simulink model "psd_project"  (R2015a)
settings: Solver=ode45  StartTime=0.0  StopTime=10  RelTol=1e-3
libraries: dsparch4 x19, dspvision x13, commchan3 x1
settings Model: Creator=aluno  LastModifiedBy=aluno

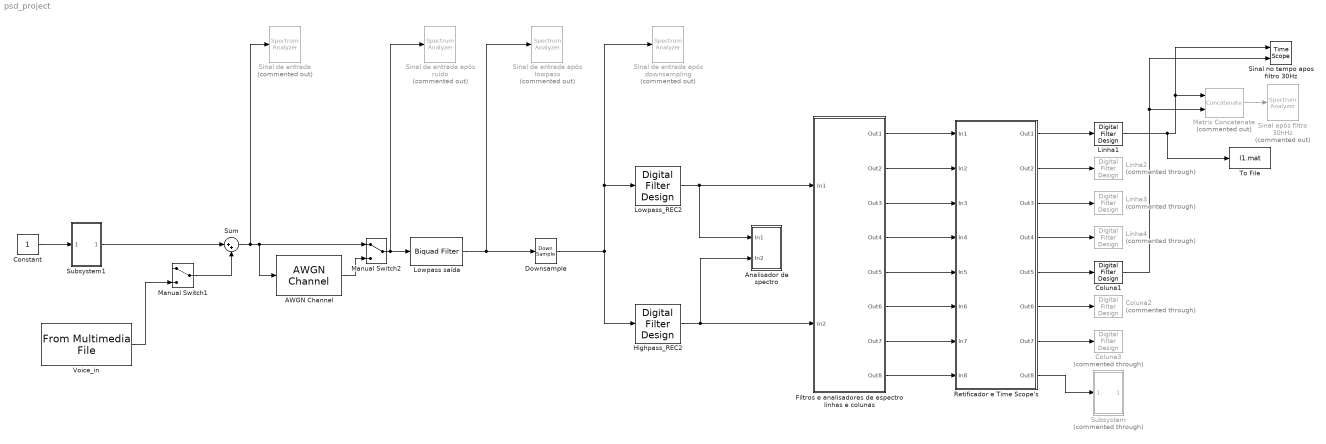
== system psd_project ==
  AWGN Channel : commchan3/AWGN Channel  InputProcessing=Columns as channels (frame based)  seed=67  noiseMode="Signal to noise ratio  (SNR)"  EbNodB=30  EsNodB=10  SNRdB=5  bitsPerSym=1  Ps=1  Tsym=1  variance=1
  Analisador de spectro : Subsystem
  Coluna1 : dsparch4/Digital Filter Design  mwdsp_browser_bugfix_var=off
  Coluna2 : dsparch4/Digital Filter Design  Commented=through  mwdsp_browser_bugfix_var=off
  Coluna3 : dsparch4/Digital Filter Design  Commented=through  mwdsp_browser_bugfix_var=off
  Constant : Constant
  Downsample : DownSample  N=11  RateOptions=Allow multirate processing
  Filtros e analisadores de espectro linhas e colunas : Subsystem
  "Highpass_REC2 " : dsparch4/Digital Filter Design  mwdsp_browser_bugfix_var=off
  Linha1 : dsparch4/Digital Filter Design  mwdsp_browser_bugfix_var=off
  Linha2 : dsparch4/Digital Filter Design  Commented=through  mwdsp_browser_bugfix_var=off
  Linha3 : dsparch4/Digital Filter Design  Commented=through  mwdsp_browser_bugfix_var=off
  Linha4 : dsparch4/Digital Filter Design  Commented=through  mwdsp_browser_bugfix_var=off
  Lowpass saída : dsparch4/Biquad Filter  Tag=BlockMethodSubSystem  IIRFiltStruct=Direct form II  CoeffSource=Specify via dialog  BiQuadCoeffs=[1 2 1 1 -1.79888261046551445 0.817336179398032825]  a0Flag=Warning  IC=0  ICnum=0  ICden=0  InputProcessing=Columns as channels (frame based)  denAccumFracLength=30  denProdOutputFracLength=30  secondMemoryFracLength=15  roundingMode=Floor  overflowMode=off  ScaleValues=[0.00461339223312960938;1]  optimizeScaleValues=on  ScaleValueMode=Specify via input port (g)  scaleValueFracLength=14  FilterSource=Specify via dialog  FilterObject=Hm_biquad
  Lowpass_REC2 : dsparch4/Digital Filter Design  mwdsp_browser_bugfix_var=off
  Manual Switch1 : ManualSwitch
  Manual Switch2 : ManualSwitch
  Matrix Concatenate : Concatenate  Commented=on  Mode=Multidimensional array  ConcatenateDimension=2
  Retificador e Time Scope's : Subsystem
  Sinal após filtro 30hHz : SpectrumAnalyzer  Commented=on
  "Sinal de entrada " : SpectrumAnalyzer  Commented=on
  "Sinal de entrada após downsampling " : SpectrumAnalyzer  Commented=on
  "Sinal de entrada após lowpass " : SpectrumAnalyzer  Commented=on
  "Sinal de entrada após ruído " : SpectrumAnalyzer  Commented=on
  Sinal no tempo apos filtro 30Hz : TimeScope  DefaultConfigurationName=spbscopes.TimeScopeBlockCfg  NumInputPorts=2
  Subsystem : Subsystem  Commented=through
  Subsystem1 : Subsystem
  Sum : Sum  Inputs=|++
  To File : ToFile  Filename=l1.mat  MatrixName=l1
  "Voice_in " : dspvision/From Multimedia File  inputFilename=/home/aluno/Projeto_Final_PSD/Audios DTMF/9-DTMF.wav  loop=on  numPlays=inf  outputStreams=Audio only  videoDataType=single  audioDataType=double  inheritSampleTime=on  userDefinedSampleTime=1/30  noAudioOutput=off  isIntensityVideo=off  fourcc=RGB  colorVideoFormat=Separate color signals  outputEOF=off  dataOrg=Column-major  audioFrameSize=1  computeAudioFrameSize=off  outSamplingMode=Sample based
  wires:
  "Voice_in "/1 -> Manual Switch1/2
  AWGN Channel/1 -> Manual Switch2/2
  Manual Switch1/1 -> Sum/2
  Lowpass saída/1 -> "Sinal de entrada após lowpass "/1, Downsample/1
  Manual Switch2/1 -> "Sinal de entrada após ruído "/1, Lowpass saída/1
  Sum/1 -> "Sinal de entrada "/1, Manual Switch2/1, AWGN Channel/1
  Lowpass_REC2/1 -> Filtros e analisadores de espectro linhas e colunas/1(In1), Analisador de spectro/1(In1)
  "Highpass_REC2 "/1 -> Analisador de spectro/2(In2), Filtros e analisadores de espectro linhas e colunas/2(In2)
  Downsample/1 -> "Highpass_REC2 "/1, Lowpass_REC2/1, "Sinal de entrada após downsampling "/1
  Filtros e analisadores de espectro linhas e colunas/1(Out1) -> Retificador e Time Scope's/1(In1)
  Filtros e analisadores de espectro linhas e colunas/2(Out2) -> Retificador e Time Scope's/2(In2)
  Filtros e analisadores de espectro linhas e colunas/3(Out3) -> Retificador e Time Scope's/3(In3)
  Filtros e analisadores de espectro linhas e colunas/4(Out4) -> Retificador e Time Scope's/4(In4)
  Filtros e analisadores de espectro linhas e colunas/5(Out5) -> Retificador e Time Scope's/5(In5)
  Filtros e analisadores de espectro linhas e colunas/6(Out6) -> Retificador e Time Scope's/6(In6)
  Filtros e analisadores de espectro linhas e colunas/7(Out7) -> Retificador e Time Scope's/7(In7)
  Filtros e analisadores de espectro linhas e colunas/8(Out8) -> Retificador e Time Scope's/8(In8)
  Retificador e Time Scope's/1(Out1) -> Linha1/1
  Retificador e Time Scope's/2(Out2) -> Linha2/1
  Retificador e Time Scope's/3(Out3) -> Linha3/1
  Retificador e Time Scope's/4(Out4) -> Linha4/1
  Retificador e Time Scope's/5(Out5) -> Coluna1/1
  Retificador e Time Scope's/6(Out6) -> Coluna2/1
  Retificador e Time Scope's/7(Out7) -> Coluna3/1
  Linha1/1 -> To File/1, Matrix Concatenate/1, Sinal no tempo apos filtro 30Hz/1
  Retificador e Time Scope's/8(Out8) -> Subsystem/1(In1)
  Matrix Concatenate/1 -> Sinal após filtro 30hHz/1
  Coluna1/1 -> Matrix Concatenate/2, Sinal no tempo apos filtro 30Hz/2
  Constant/1 -> Subsystem1/1(In1)
  Subsystem1/1(Out1) -> Sum/1

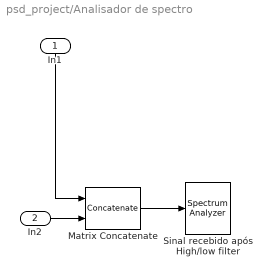
== system psd_project/Analisador de spectro ==
  In1 : Inport
  In2 : Inport  Port=2
  Matrix Concatenate : Concatenate  Mode=Multidimensional array  ConcatenateDimension=2
  Sinal recebido após High/low filter : SpectrumAnalyzer
  wires:
  In1/1 -> Matrix Concatenate/1
  In2/1 -> Matrix Concatenate/2
  Matrix Concatenate/1 -> Sinal recebido após High/low filter/1

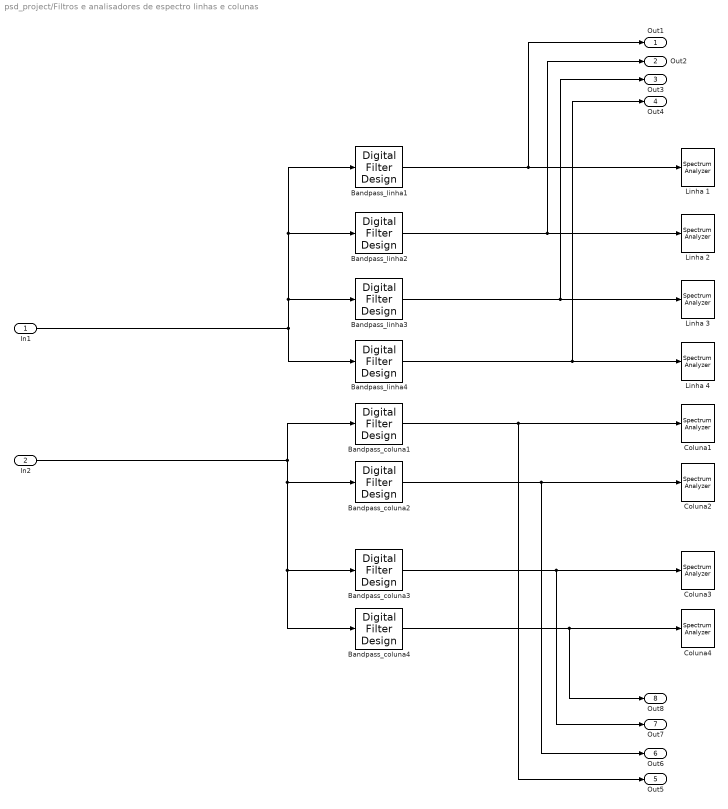
== system psd_project/Filtros e analisadores de espectro linhas e colunas ==
  In1 : Inport
  In2 : Inport  Port=2
  Bandpass_coluna{1..4} (4 alike) : dsparch4/Digital Filter Design  mwdsp_browser_bugfix_var=off
  Bandpass_linha{1..4} (4 alike) : dsparch4/Digital Filter Design  mwdsp_browser_bugfix_var=off
  "Coluna1 " : SpectrumAnalyzer
  "Coluna2 " : SpectrumAnalyzer
  Coluna3 : SpectrumAnalyzer
  Coluna4 : SpectrumAnalyzer
  Linha {1..4} (4 alike) : SpectrumAnalyzer
  Out1 : Outport
  Out2 : Outport  Port=2
  Out3 : Outport  Port=3
  Out4 : Outport  Port=4
  Out5 : Outport  Port=5
  Out6 : Outport  Port=6
  Out7 : Outport  Port=7
  Out8 : Outport  Port=8
  wires:
  In1/1 -> Bandpass_linha4/1, Bandpass_linha3/1, Bandpass_linha2/1, Bandpass_linha1/1
  In2/1 -> Bandpass_coluna1/1, Bandpass_coluna2/1, Bandpass_coluna4/1, Bandpass_coluna3/1
  Bandpass_linha1/1 -> Out1/1, Linha 1/1
  Bandpass_linha4/1 -> Out4/1, Linha 4/1
  Bandpass_linha2/1 -> Out2/1, Linha 2/1
  Bandpass_coluna3/1 -> Out7/1, Coluna3/1
  Bandpass_coluna2/1 -> Out6/1, "Coluna2 "/1
  Bandpass_coluna4/1 -> Out8/1, Coluna4/1
  Bandpass_linha3/1 -> Out3/1, Linha 3/1
  Bandpass_coluna1/1 -> Out5/1, "Coluna1 "/1

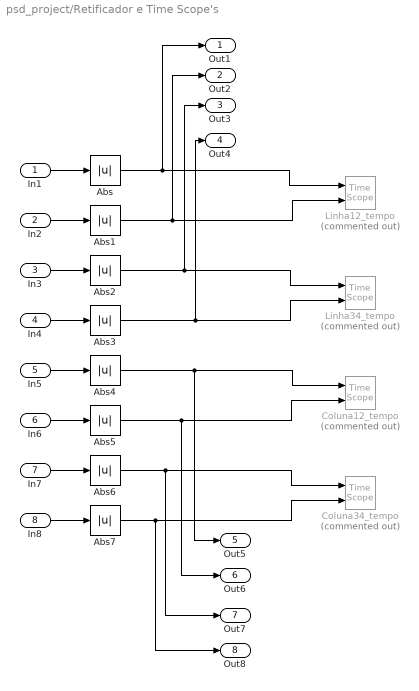
== system psd_project/Retificador e Time Scope's ==
  In1 : Inport
  In2 : Inport  Port=2
  In3 : Inport  Port=3
  In4 : Inport  Port=4
  In5 : Inport  Port=5
  In6 : Inport  Port=6
  In7 : Inport  Port=7
  In8 : Inport  Port=8
  Abs{,1..7} (8 alike) : Abs
  Coluna12_tempo : TimeScope  Commented=on  DefaultConfigurationName=spbscopes.TimeScopeBlockCfg  NumInputPorts=2
  Coluna34_tempo : TimeScope  Commented=on  DefaultConfigurationName=spbscopes.TimeScopeBlockCfg  NumInputPorts=2
  "Linha12_tempo " : TimeScope  Commented=on  DefaultConfigurationName=spbscopes.TimeScopeBlockCfg  NumInputPorts=2
  Linha34_tempo : TimeScope  Commented=on  DefaultConfigurationName=spbscopes.TimeScopeBlockCfg  NumInputPorts=2
  Out1 : Outport
  Out2 : Outport  Port=2
  Out3 : Outport  Port=3
  Out4 : Outport  Port=4
  Out5 : Outport  Port=5
  Out6 : Outport  Port=6
  Out7 : Outport  Port=7
  Out8 : Outport  Port=8
  wires:
  Abs6/1 -> Out7/1, Coluna34_tempo/1
  Abs5/1 -> Coluna12_tempo/2, Out6/1
  Abs4/1 -> Out5/1, Coluna12_tempo/1
  Abs2/1 -> Out3/1, Linha34_tempo/1
  Abs7/1 -> Out8/1, Coluna34_tempo/2
  Abs3/1 -> Out4/1, Linha34_tempo/2
  In6/1 -> Abs5/1
  In3/1 -> Abs2/1
  In4/1 -> Abs3/1
  In2/1 -> Abs1/1
  Abs1/1 -> Out2/1, "Linha12_tempo "/2
  In7/1 -> Abs6/1
  Abs/1 -> Out1/1, "Linha12_tempo "/1
  In5/1 -> Abs4/1
  In8/1 -> Abs7/1
  In1/1 -> Abs/1

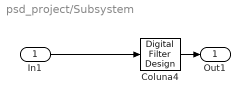
== system psd_project/Subsystem ==
  In1 : Inport
  Coluna4 : dsparch4/Digital Filter Design  mwdsp_browser_bugfix_var=off
  Out1 : Outport
  wires:
  Coluna4/1 -> Out1/1
  In1/1 -> Coluna4/1

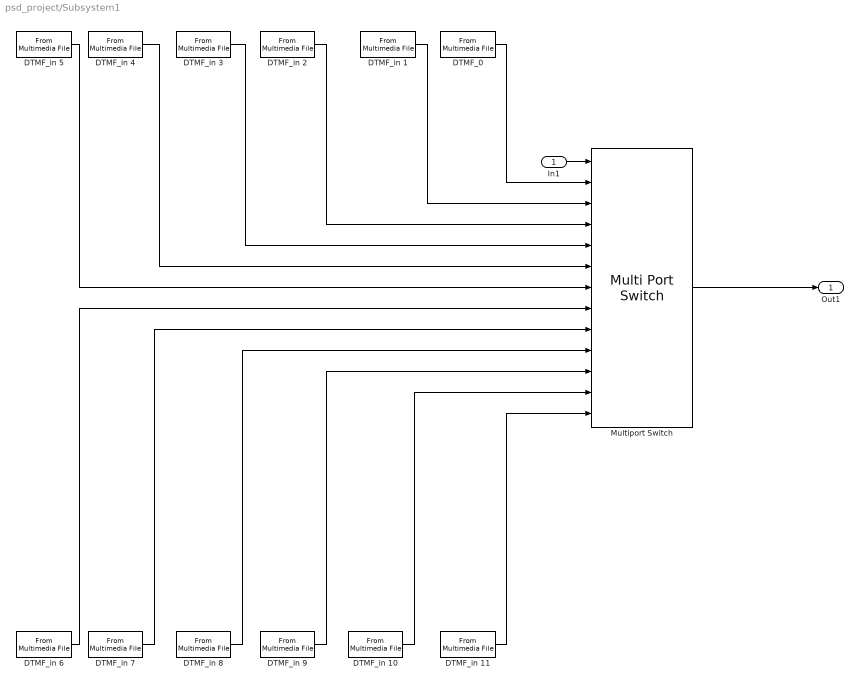
== system psd_project/Subsystem1 ==
  In1 : Inport
  "DTMF_0 " : dspvision/From Multimedia File  inputFilename=/home/aluno/Projeto_Final_PSD/Audios DTMF com Pausa/0-DTMF.wav  loop=on  numPlays=inf  outputStreams=Audio only  videoDataType=single  audioDataType=double  inheritSampleTime=on  userDefinedSampleTime=1/30  noAudioOutput=off  isIntensityVideo=off  fourcc=RGB  colorVideoFormat=Separate color signals  outputEOF=off  dataOrg=Column-major  audioFrameSize=1  computeAudioFrameSize=off  outSamplingMode=Sample based
  DTMF_in 1 : dspvision/From Multimedia File  inputFilename=/home/aluno/Projeto_Final_PSD/Audios DTMF com Pausa/1-DTMF.wav  loop=on  numPlays=inf  outputStreams=Audio only  videoDataType=single  audioDataType=double  inheritSampleTime=on  userDefinedSampleTime=1/30  noAudioOutput=off  isIntensityVideo=off  fourcc=RGB  colorVideoFormat=Separate color signals  outputEOF=off  dataOrg=Column-major  audioFrameSize=1  computeAudioFrameSize=off  outSamplingMode=Sample based
  DTMF_in 10 : dspvision/From Multimedia File  inputFilename=/home/aluno/Projeto_Final_PSD/Audios DTMF com Pausa/asterisk-DTMF.wav  loop=on  numPlays=inf  outputStreams=Audio only  videoDataType=single  audioDataType=double  inheritSampleTime=on  userDefinedSampleTime=1/30  noAudioOutput=off  isIntensityVideo=off  fourcc=RGB  colorVideoFormat=Separate color signals  outputEOF=off  dataOrg=Column-major  audioFrameSize=1  computeAudioFrameSize=off  outSamplingMode=Sample based
  DTMF_in 11 : dspvision/From Multimedia File  inputFilename=/home/aluno/Projeto_Final_PSD/Audios DTMF com Pausa/#-DTMF.wav  loop=on  numPlays=inf  outputStreams=Audio only  videoDataType=single  audioDataType=double  inheritSampleTime=on  userDefinedSampleTime=1/30  noAudioOutput=off  isIntensityVideo=off  fourcc=RGB  colorVideoFormat=Separate color signals  outputEOF=off  dataOrg=Column-major  audioFrameSize=1  computeAudioFrameSize=off  outSamplingMode=Sample based
  DTMF_in 2 : dspvision/From Multimedia File  inputFilename=/home/aluno/Projeto_Final_PSD/Audios DTMF com Pausa/2-DTMF.wav  loop=on  numPlays=inf  outputStreams=Audio only  videoDataType=single  audioDataType=double  inheritSampleTime=on  userDefinedSampleTime=1/30  noAudioOutput=off  isIntensityVideo=off  fourcc=RGB  colorVideoFormat=Separate color signals  outputEOF=off  dataOrg=Column-major  audioFrameSize=1  computeAudioFrameSize=off  outSamplingMode=Sample based
  DTMF_in 3 : dspvision/From Multimedia File  inputFilename=/home/aluno/Projeto_Final_PSD/Audios DTMF com Pausa/3-DTMF.wav  loop=on  numPlays=inf  outputStreams=Audio only  videoDataType=single  audioDataType=double  inheritSampleTime=on  userDefinedSampleTime=1/30  noAudioOutput=off  isIntensityVideo=off  fourcc=RGB  colorVideoFormat=Separate color signals  outputEOF=off  dataOrg=Column-major  audioFrameSize=1  computeAudioFrameSize=off  outSamplingMode=Sample based
  DTMF_in 4 : dspvision/From Multimedia File  inputFilename=/home/aluno/Projeto_Final_PSD/Audios DTMF com Pausa/4-DTMF.wav  loop=on  numPlays=inf  outputStreams=Audio only  videoDataType=single  audioDataType=double  inheritSampleTime=on  userDefinedSampleTime=1/30  noAudioOutput=off  isIntensityVideo=off  fourcc=RGB  colorVideoFormat=Separate color signals  outputEOF=off  dataOrg=Column-major  audioFrameSize=1  computeAudioFrameSize=off  outSamplingMode=Sample based
  DTMF_in 5 : dspvision/From Multimedia File  inputFilename=/home/aluno/Projeto_Final_PSD/Audios DTMF com Pausa/5-DTMF.wav  loop=on  numPlays=inf  outputStreams=Audio only  videoDataType=single  audioDataType=double  inheritSampleTime=on  userDefinedSampleTime=1/30  noAudioOutput=off  isIntensityVideo=off  fourcc=RGB  colorVideoFormat=Separate color signals  outputEOF=off  dataOrg=Column-major  audioFrameSize=1  computeAudioFrameSize=off  outSamplingMode=Sample based
  DTMF_in 6 : dspvision/From Multimedia File  inputFilename=/home/aluno/Projeto_Final_PSD/Audios DTMF com Pausa/6-DTMF.wav  loop=on  numPlays=inf  outputStreams=Audio only  videoDataType=single  audioDataType=double  inheritSampleTime=on  userDefinedSampleTime=1/30  noAudioOutput=off  isIntensityVideo=off  fourcc=RGB  colorVideoFormat=Separate color signals  outputEOF=off  dataOrg=Column-major  audioFrameSize=1  computeAudioFrameSize=off  outSamplingMode=Sample based
  DTMF_in 7 : dspvision/From Multimedia File  inputFilename=/home/aluno/Projeto_Final_PSD/Audios DTMF com Pausa/7-DTMF.wav  loop=on  numPlays=inf  outputStreams=Audio only  videoDataType=single  audioDataType=double  inheritSampleTime=on  userDefinedSampleTime=1/30  noAudioOutput=off  isIntensityVideo=off  fourcc=RGB  colorVideoFormat=Separate color signals  outputEOF=off  dataOrg=Column-major  audioFrameSize=1  computeAudioFrameSize=off  outSamplingMode=Sample based
  DTMF_in 8 : dspvision/From Multimedia File  inputFilename=/home/aluno/Projeto_Final_PSD/Audios DTMF com Pausa/8-DTMF.wav  loop=on  numPlays=inf  outputStreams=Audio only  videoDataType=single  audioDataType=double  inheritSampleTime=on  userDefinedSampleTime=1/30  noAudioOutput=off  isIntensityVideo=off  fourcc=RGB  colorVideoFormat=Separate color signals  outputEOF=off  dataOrg=Column-major  audioFrameSize=1  computeAudioFrameSize=off  outSamplingMode=Sample based
  DTMF_in 9 : dspvision/From Multimedia File  inputFilename=/home/aluno/Projeto_Final_PSD/Audios DTMF com Pausa/9-DTMF.wav  loop=on  numPlays=inf  outputStreams=Audio only  videoDataType=single  audioDataType=double  inheritSampleTime=on  userDefinedSampleTime=1/30  noAudioOutput=off  isIntensityVideo=off  fourcc=RGB  colorVideoFormat=Separate color signals  outputEOF=off  dataOrg=Column-major  audioFrameSize=1  computeAudioFrameSize=off  outSamplingMode=Sample based
  Multiport Switch : MultiPortSwitch  DataPortOrder=Specify indices  Inputs=12  DataPortIndices={0,1,2,3,4,5,6,7,8,9,10,11}
  Out1 : Outport
  wires:
  DTMF_in 7/1 -> Multiport Switch/9
  Multiport Switch/1 -> Out1/1
  DTMF_in 3/1 -> Multiport Switch/5
  DTMF_in 5/1 -> Multiport Switch/7
  DTMF_in 8/1 -> Multiport Switch/10
  In1/1 -> Multiport Switch/1
  DTMF_in 1/1 -> Multiport Switch/3
  DTMF_in 4/1 -> Multiport Switch/6
  DTMF_in 9/1 -> Multiport Switch/11
  DTMF_in 10/1 -> Multiport Switch/12
  DTMF_in 2/1 -> Multiport Switch/4
  DTMF_in 6/1 -> Multiport Switch/8
  "DTMF_0 "/1 -> Multiport Switch/2
  DTMF_in 11/1 -> Multiport Switch/13
